simulink model "Example_IOBlock_Library_CCP"  (Simulink 10.3)
settings: Solver=FixedStepDiscrete  StartTime=0.0  StopTime=10.0  FixedStep=0.01  RelTol=1e-3
model workspace (MAT data in the model file):
  ParameterA_CCP_Test = Simulink.Parameter
  ParameterA_CCP_Test.Value = 23456
  ParameterA_CCP_Test.DataType = 'uint16'
  ParameterA_CCP_Test.Dimensions = [1 1]
  ParameterB_CCP_Test = Simulink.Parameter
  ParameterB_CCP_Test.Value = 0.5
  ParameterB_CCP_Test.DataType = 'single'
  ParameterB_CCP_Test.Min = 0
  ParameterB_CCP_Test.Max = 10
  ParameterB_CCP_Test.Dimensions = [1 1]
libraries: IOBlock_Library_TTC580 x9, AddOn_Lib_TTC580_CCP x2
settings Model: Creator=hokka  LastModifiedBy=hokka  MultithreadedSim=on
settings Model: SuppressorTable=|
  | <?xml version="1.0" encoding="UTF-8" standalone="yes" ?>
  | <!DOCTYPE boost_serialization>
  | <boost_serialization signature="serialization::archive" version="17">
  | <DiagnosticSuppressor class_id="0" tracking_level="0" version="7">
  | 	<Table class_id="1" tracking_level="0" version="0">
  | 		<count>7</count>
  | 		<bucket_count>8</bucket_count>
  | 		<item_version>0</item_version>
  | 		<item class_id="2" tracking_level="0" version="0">
  | 			<first class_id="3" tracking_level="0" version="7">
  | 				<Source class_id="4" tracking_level="0" version="0">
  | 					<count>1</count>
  | 					<item_version>0</item_version>
  | 					<item>74:2245</item>
  | 				</Source>
  | 			</first>
  | 			<second class_id="5" tracking_level="0" version="7">
  | 				<SuppressedData class_id="6" tracking_level="0" version="0">
  | 					<count>2</count>
  | 					<bucket_count>8</bucket_count>
  | 					<item_version>0</item_version>
  | 					<item class_id="7" tracking_level="0" version="0">
  | 						<first class_id="8" tracking_level="0" version="7">
  | 							<ID>Simulink:DataType:WarningOverFlowDetected</ID>
  | 							<Cause>
  | 								<Source>
  | 									<count>0</count>
  | 									<item_version>0</item_version>
  | 								</Source>
  | 							</Cause>
  | 						</first>
  | 						<second class_id="9" tracking_level="0" version="7">
  | 							<Comment></Comment>
  | 							<User></User>
  | 							<LastModified class_id="10" tracking_level="0" version="0">
  | 								<ptime_date class_id="11" tracking_level="0" version="0">
  | 									<date>20160608</date>
  | 								</ptime_date>
  | 								<ptime_time_duration class_id="12" tracking_level="0" version="1">
  | 									<is_special>0</is_special>
  | 									<time_duration_hours>15</time_duration_hours>
  | 									<time_duration_minutes>23</time_duration_minutes>
  | 									<time_duration_seconds>17</time_duration_seconds>
  | 									<time_duration_fractional_seconds>0</time_duration_fractional_seconds>
  | 								</ptime_time_duration>
  | 							</LastModified>
  | 							<SuppressionType>1</SuppressionType>
  | 						</second>
  | 					</item>
  | 					<item>
  | 						<first>
  | 							<ID>SimulinkFixedPoint:util:Overflowoccurred</ID>
  | 							<Cause>
  | 								<Source>
  | 									<count>0</count>
  | 									<item_version>0</item_version>
  | 								</Source>
  | 							</Cause>
  | 						</first>
  | 						<second>
  | 							<Comment></Comment>
  | 							<User></User>
  | 							<LastModified>
  | 								<ptime_date>
  | 									<date>20160608</date>
  | 								</ptime_date>
  | 								<ptime_time_duration>
  | 									<is_special>0</is_special>
  | 									<time_duration_hours>15</time_duration_hours>
  | 									<time_duration_minutes>23</time_duration_minutes>
  | 									<time_duration_seconds>17</time_duration_seconds>
  | 									<time_duration_fractional_seconds>0</time_duration_fractional_seconds>
  | 								</ptime_time_duration>
  | 							</LastModified>
  | 							<SuppressionType>1</SuppressionType>
  | 						</second>
  | 					</item>
  | 				</SuppressedData>
  | 			</second>
  | 		</item>
  | 		<item>
  | 			<first>
  | 				<Source>
  | 					<count>1</count>
  | 					<item_version>0</item_version>
  | 					<item>38:2245</item>
  | 				</Source>
  | 			</first>
  | 			<second>
  | 				<SuppressedData>
  | 					<count>2</count>
  | 					<bucket_count>8</bucket_count>
  | 					<item_version>0</item_version>
  | 					<item>
  | 						<first>
  | 							<ID>Simulink:DataType:WarningOverFlowDetected</ID>
  | 							<Cause>
  | 								<Source>
  | 									<count>0</count>
  | 									<item_version>0</item_version>
  | 								</Source>
  | 							</Cause>
  | 						</first>
  | 						<second>
  | 							<Comment></Comment>
  | 							<User></User>
  | 							<LastModified>
  | 								<ptime_date>
  | 									<date>20160608</date>
  | 								</ptime_date>
  | 								<ptime_time_duration>
  | 									<is_special>0</is_special>
  | 									<time_duration_hours>15</time_duration_hours>
  | 									<time_duration_minutes>23</time_duration_minutes>
  | 									<time_duration_seconds>17</time_duration_seconds>
  | 									<time_duration_fractional_seconds>0</time_duration_fractional_seconds>
  | 								</ptime_time_duration>
  | 							</LastModified>
  | 							<SuppressionType>1</SuppressionType>
  | 						</second>
  | 					</item>
  | 					<item>
  | 						<first>
  | 							<ID>SimulinkFixedPoint:util:Overflowoccurred</ID>
  | 							<Cause>
  | 								<Source>
  | 									<count>0</count>
  | 									<item_version>0</item_version>
  | 								</Source>
  | 							</Cause>
  | 						</first>
  | 						<second>
  | 							<Comment></Comment>
  | 							<User></User>
  | 							<LastModified>
  | 								<ptime_date>
  | 									<date>20160608</date>
  | 								</ptime_date>
  | 								<ptime_time_duration>
  | 									<is_special>0</is_special>
  | 									<time_duration_hours>15</time_duration_hours>
  | 									<time_duration_minutes>23</time_duration_minutes>
  | 									<time_duration_seconds>17</time_duration_seconds>
  | 									<time_duration_fractional_seconds>0</time_duration_fractional_seconds>
  | 								</ptime_time_duration>
  | 							</LastModified>
  | 							<SuppressionType>1</SuppressionType>
  | 						</second>
  | 					</item>
  | 				</SuppressedData>
  | 			</second>
  | 		</item>
  | 		<item>
  | 			<first>
  | 				<Source>
  | 					<count>1</count>
  | 					<item_version>0</item_version>
  | 					<item>23:2245</item>
  | 				</Source>
  | 			</first>
  | 			<second>
  | 				<SuppressedData>
  | 					<count>2</count>
  | 					<bucket_count>8</bucket_count>
  | 					<item_version>0</item_version>
  | 					<item>
  | 						<first>
  | 							<ID>Simulink:DataType:WarningOverFlowDetected</ID>
  | 							<Cause>
  | 								<Source>
  | 									<count>0</count>
  | 									<item_version>0</item_version>
  | 								</Source>
  | 							</Cause>
  | 						</first>
  | 						<second>
  | 							<Comment></Comment>
  | 							<User></User>
  | 							<LastModified>
  | 								<ptime_date>
  | 									<date>20160608</date>
  | 								</ptime_date>
  | 								<ptime_time_duration>
  | 									<is_special>0</is_special>
  | 									<time_duration_hours>15</time_duration_hours>
  | 									<time_duration_minutes>23</time_duration_minutes>
  | 									<time_duration_seconds>17</time_duration_seconds>
  | 									<time_duration_fractional_seconds>0</time_duration_fractional_seconds>
  | 								</ptime_time_duration>
  | 							</LastModified>
  | 							<SuppressionType>1</SuppressionType>
  | 						</second>
  | 					</item>
  | 					<item>
  | 						<first>
  | 							<ID>SimulinkFixedPoint:util:Overflowoccurred</ID>
  | 							<Cause>
  | 								<Source>
  | 									<count>0</count>
  | 									<item_version>0</item_version>
  | 								</Source>
  | 							</Cause>
  | 						</first>
  | 						<second>
  | 							<Comment></Comment>
  | 							<User></User>
  | 							<LastModified>
  | 								<ptime_date>
  | 									<date>20160608</date>
  | 								</ptime_date>
  | 								<ptime_time_duration>
  | 									<is_special>0</is_special>
  | 									<time_duration_hours>15</time_duration_hours>
  | 									<time_duration_minutes>23</time_duration_minutes>
  | 									<time_duration_seconds>17</time_duration_seconds>
  | 									<time_duration_fractional_seconds>0</time_duration_fractional_seconds>
  | 								</ptime_time_duration>
  | 							</LastModified>
  | 							<SuppressionType>1</SuppressionType>
  | 						</second>
  | 					</item>
  | 				</SuppressedData>
  | 			</second>
  | 		</item>
  | 		<item>
  | 			<first>
  | 				<Source>
  | 					<count>1</count>
  | 					<item_version>0</item_version>
  | 					<item>39:2245</item>
  | 				</Source>
  | 			</first>
  | 			<second>
  | 				<SuppressedData>
  | 					<count>2</count>
  | 					<bucket_count>8</bucket_count>
  | 					<item_version>0</item_version>
  | 					<item>
  | 						<first>
  | 							<ID>Simulink:DataType:WarningOverFlowDetected</ID>
  | 							<Cause>
  | 								<Source>
  | 									<count>0</count>
  | 									<item_version>0</item_version>
  | 								</Source>
  | 							</Cause>
  | 						</first>
  | 						<second>
  | 							<Comment></Comment>
  | 							<User></User>
  | 							<LastModified>
  | 								<ptime_date>
  | 									<date>20160608</date>
  | 								</ptime_date>
  | 								<ptime_time_duration>
  | 									<is_special>0</is_special>
  | 									<time_duration_hours>15</time_duration_hours>
  | 									<time_duration_minutes>23</time_duration_minutes>
  | 									<time_duration_seconds>17</time_duration_seconds>
  | 									<time_duration_fractional_seconds>0</time_duration_fractional_seconds>
  | 								</ptime_time_duration>
  | 							</LastModified>
  | 							<SuppressionType>1</SuppressionType>
  | 						</second>
  | 					</item>
  | 					<item>
  | 						<first>
  | 							<ID>SimulinkFixedPoint:util:Overflowoccurred</ID>
  | 							<Cause>
  | 								<Source>
  | 									<count>0</count>
  | 									<item_version>0</item_version>
  | 								</Source>
  | 							</Cause>
  | 						</first>
  | 						<second>
  | 							<Comment></Comment>
  | 							<User></User>
  | 							<LastModified>
  | 								<ptime_date>
  | 									<date>20160608</date>
  | 								</ptime_date>
  | 								<ptime_time_duration>
  | 									<is_special>0</is_special>
  | 									<time_duration_hours>15</time_duration_hours>
  | 									<time_duration_minutes>23</time_duration_minutes>
  | 									<time_duration_seconds>17</time_duration_seconds>
  | 									<time_duration_fractional_seconds>0</time_duration_fractional_seconds>
  | 								</ptime_time_duration>
  | 							</LastModified>
  | 							<SuppressionType>1</SuppressionType>
  | 						</second>
  | 					</item>
  | 				</SuppressedData>
  | 			</second>
  | 		</item>
  | 		<item>
  | 			<first>
  | 				<Source>
  | 					<count>1</count>
  | 					<item_version>0</item_version>
  | 					<item>103:2245</item>
  | 				</Source>
  | 			</first>
  | 			<second>
  | 				<SuppressedData>
  | 					<count>2</count>
  | 					<bucket_count>8</bucket_count>
  | 					<item_version>0</item_version>
  | 					<item>
  | 						<first>
  | 							<ID>Simulink:DataType:WarningOverFlowDetected</ID>
  | 							<Cause>
  | 								<Source>
  | 									<count>0</count>
  | 									<item_version>0</item_version>
  | 								</Source>
  | 							</Cause>
  | 						</first>
  | 						<second>
  | 							<Comment></Comment>
  | 							<User></User>
  | 							<LastModified>
  | 								<ptime_date>
  | 									<date>20160608</date>
  | 								</ptime_date>
  | 								<ptime_time_duration>
  | 									<is_special>0</is_special>
  | 									<time_duration_hours>15</time_duration_hours>
  | 									<time_duration_minutes>23</time_duration_minutes>
  | 									<time_duration_seconds>17</time_duration_seconds>
  | 									<time_duration_fractional_seconds>0</time_duration_fractional_seconds>
  | 								</ptime_time_duration>
  | 							</LastModified>
  | 							<SuppressionType>1</SuppressionType>
  | 						</second>
  | 					</item>
  | 					<item>
  | 						<first>
  | 							<ID>SimulinkFixedPoint:util:Overflowoccurred</ID>
  | 							<Cause>
  | 								<Source>
  | 									<count>0</count>
  | 									<item_version>0</item_version>
  | 								</Source>
  | 							</Cause>
  | 						</first>
  | 						<second>
  | 							<Comment></Comment>
  | 							<User></User>
  | 							<LastModified>
  | 								<ptime_date>
  | 									<date>20160608</date>
  | 								</ptime_date>
  | 								<ptime_time_duration>
  | 									<is_special>0</is_special>
  | 									<time_duration_hours>15</time_duration_hours>
  | 									<time_duration_minutes>23</time_duration_minutes>
  | 									<time_duration_seconds>17</time_duration_seconds>
  | 									<time_duration_fractional_seconds>0</time_duration_fractional_seconds>
  | 								</ptime_time_duration>
  | 							</LastModified>
  | 							<SuppressionType>1</SuppressionType>
  | 						</second>
  | 					</item>
  | 				</SuppressedData>
  | 			</second>
  | 		</item>
  | 		<item>
  | 			<first>
  | 				<Source>
  | 					<count>1</count>
  | 					<item_version>0</item_version>
  | 					<item>40:2245</item>
  | 				</Source>
  | 			</first>
  | 			<second>
  | 				<SuppressedData>
  | 					<count>2</count>
  | 					<bucket_count>8</bucket_count>
  | 					<item_version>0</item_version>
  | 					<item>
  | 						<first>
  | 							<ID>Simulink:DataType:WarningOverFlowDetected</ID>
  | 							<Cause>
  | 								<Source>
  | 									<count>0</count>
  | 									<item_version>0</item_version>
  | 								</Source>
  | 							</Cause>
  | 						</first>
  | 						<second>
  | 							<Comment></Comment>
  | 							<User></User>
  | 							<LastModified>
  | 								<ptime_date>
  | 									<date>20160608</date>
  | 								</ptime_date>
  | 								<ptime_time_duration>
  | 									<is_special>0</is_special>
  | 									<time_duration_hours>15</time_duration_hours>
  | 									<time_duration_minutes>23</time_duration_minutes>
  | 									<time_duration_seconds>17</time_duration_seconds>
  | 									<time_duration_fractional_seconds>0</time_duration_fractional_seconds>
  | 								</ptime_time_duration>
  | 							</LastModified>
  | 							<SuppressionType>1</SuppressionType>
  | 						</second>
  | 					</item>
  | 					<item>
  | 						<first>
  | 							<ID>SimulinkFixedPoint:util:Overflowoccurred</ID>
  | 							<Cause>
  | 								<Source>
  | 									<count>0</count>
  | 									<item_version>0</item_version>
  | 								</Source>
  | 							</Cause>
  | 						</first>
  | 						<second>
  | 							<Comment></Comment>
  | 							<User></User>
  | 							<LastModified>
  | 								<ptime_date>
  | 									<date>20160608</date>
  | 								</ptime_date>
  | 								<ptime_time_duration>
  | 									<is_special>0</is_special>
  | 									<time_duration_hours>15</time_duration_hours>
  | 									<time_duration_minutes>23</time_duration_minutes>
  | 									<time_duration_seconds>17</time_duration_seconds>
  | 									<time_duration_fractional_seconds>0</time_duration_fractional_seconds>
  | 								</ptime_time_duration>
  | 							</LastModified>
  | 							<SuppressionType>1</SuppressionType>
  | 						</second>
  | 					</item>
  | 				</SuppressedData>
  | 			</second>
  | 		</item>
  | 		<item>
  | 			<first>
  | 				<Source>
  | 					<count>1</count>
  | 					<item_version>0</item_version>
  | 					<item>36:2245</item>
  | 				</Source>
  | 			</first>
  | 			<second>
  | 				<SuppressedData>
  | 					<count>2</count>
  | 					<bucket_count>8</bucket_count>
  | 					<item_version>0</item_version>
  | 					<item>
  | 						<first>
  | 							<ID>Simulink:DataType:WarningOverFlowDetected</ID>
  | 							<Cause>
  | 								<Source>
  | 									<count>0</count>
  | 									<item_version>0</item_version>
  | 								</Source>
  | 							</Cause>
  | 						</first>
  | 						<second>
  | 							<Comment></Comment>
  | 							<User></User>
  | 							<LastModified>
  | 								<ptime_date>
  | 									<date>20160608</date>
  | 								</ptime_date>
  | 								<ptime_time_duration>
  | 									<is_special>0</is_special>
  | 									<time_duration_hours>15</time_duration_hours>
  | 									<time_duration_minutes>23</time_duration_minutes>
  | 									<time_duration_seconds>17</time_duration_seconds>
  | 									<time_duration_fractional_seconds>0</time_duration_fractional_seconds>
  | 								</ptime_time_duration>
  | 							</LastModified>
  | 							<SuppressionType>1</SuppressionType>
  | 						</second>
  | 					</item>
  | 					<item>
  | 						<first>
  | 							<ID>SimulinkFixedPoint:util:Overflowoccurred</ID>
  | 							<Cause>
  | 								<Source>
  | 									<count>0</count>
  | 									<item_version>0</item_version>
  | 								</Source>
  | 							</Cause>
  | 						</first>
  | 						<second>
  | 							<Comment></Comment>
  | 							<User></User>
  | 							<LastModified>
  | 								<ptime_date>
  | 									<date>20160608</date>
  | 								</ptime_date>
  | 								<ptime_time_duration>
  | 									<is_special>0</is_special>
  | 									<time_duration_hours>15</time_duration_hours>
  | 									<time_duration_minutes>23</time_duration_minutes>
  | 									<time_duration_seconds>17</time_duration_seconds>
  | 									<time_duration_fractional_seconds>0</time_duration_fractional_seconds>
  | 								</ptime_time_duration>
  | 							</LastModified>
  | 							<SuppressionType>1</SuppressionType>
  | 						</second>
  | 					</item>
  | 				</SuppressedData>
  | 			</second>
  | 		</item>
  | 	</Table>
  | </DiagnosticSuppressor>
  | 
  | </boost_serialization>
  | 
  | </boost_serialization>
settings DataIOCC: LimitDataPoints=on
settings OptimizationCC: InitFltsAndDblsToZero=on  LifeSpan=1  EfficientTunableParamExpr=on
settings DebuggingCC: SolverPrmCheckMsg=warning  InheritedTsInSrcMsg=none
settings HardwareCC: ProdLargestAtomicInteger=Long  ProdLargestAtomicFloat=Double  ProdIntDivRoundTo=Zero  ProdEndianess=BigEndian  ProdHWDeviceType=Texas Instruments->TMS570 Cortex-R4  TargetIntDivRoundTo=Zero  TargetEndianess=BigEndian  TargetHWDeviceType=Generic->32-bit Embedded Processor
settings SFSimCC: MATLABDynamicMemAlloc=off
settings RTWCC: Description=Real-Time Workshop Embedded Coder (no auto configuration)  SystemTargetFile=ert.tlc  GenCodeOnly=on  TemplateMakefile=ert_TTC580.tmf
settings CodeAppCC: IgnoreCustomStorageClasses=off  CustomSymbolStrType=$N$R$M  InternalIdentifier=Classic
settings ERTTargetCC: MultiwordLength=2048  SupportAbsoluteTime=off  SupportNonFinite=off  GenerateASAP2=on  ERTCustomFileTemplate=example_file_process.tlc  ConvertIfToSwitch=off  SuppressUnreachableDefaultCases=off
settings ConfigComp: CovSFcnEnable=off

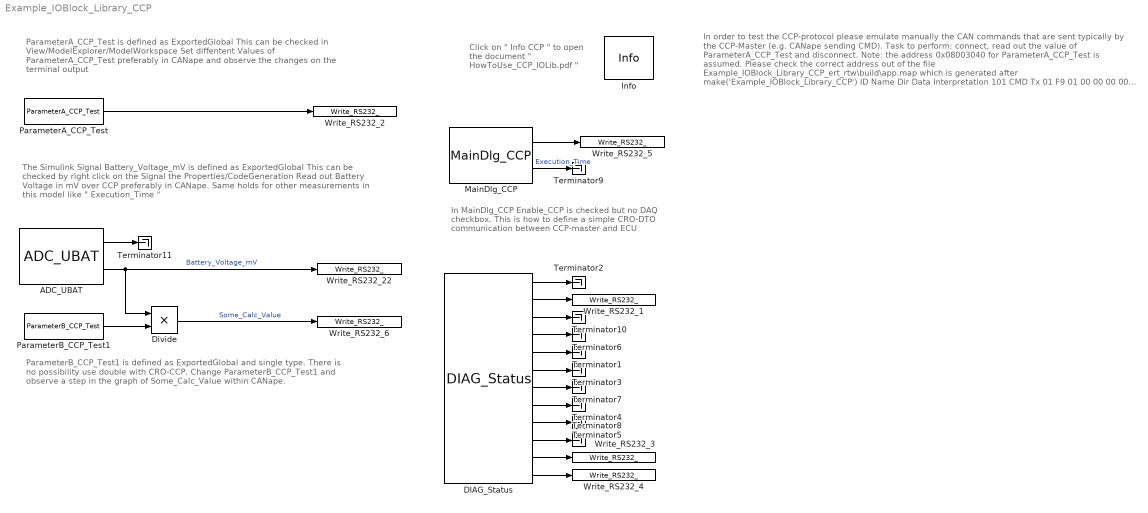
== system Example_IOBlock_Library_CCP ==
  note: In order to test the CCP-protocol please emulate manually the CAN commands that are sent typically by the CCP-Master (e.g. CANape sending CMD).
      |
      | Task to perform: connect, read out the value of ParameterA_CCP_Test and disconnect.
      |
      | Note: the address 0x08003040 for ParameterA_CCP_Test is assumed. Please check the correct address out of
      | the file Example_IOBlock_Library_CCP_ert_rtw\build\app.map which is generated after make('Example_IOBlock_Library_CCP')
      |
      | ID	Name	       Dir	Data	                Interpretation
      | 101	CMD		Tx	01 F9 01 00 00 00 00 00	CONNECT addr=0001h (CCP station addr.)
      | 102	RES		Rx	FF 00 F9 00 01 00 00 00	Ok:CONNECT
      | 101	CMD		Tx	17 FA 00 00 00 00 00 00	EXCHANGE_ID
      | 102	RES		Rx	FF 00 FA 08 00 01 00 8E	Ok:EXCHANGE_ID size=8 type=00h avail=01h protect=00h
      | 101	CMD		Tx	1B FB 02 01 00 00 00 00	GET_CCP_VERSION version=02h release=01h
      | 102	RES		Rx	FF 00 FB 02 01 01 00 8E	Ok:GET_CCP_VERSION version=02h release=01h
      | 101	CMD		Tx	0F FC 02 00 08 00 30 40	SHORT_UPLOAD size=2 ext=00h addr=08003040h
      | 102	RES		Rx	FF 00 FC 5B A0 01 00 8E	Ok:SHORT_UPLOAD data=5Bh A0h (decimal value=23456)
      | 101	CMD		Tx	07 FD 01 01 00 00  00 00	DISCONNECT addr=0001h (CCP station addr)
      | 102	RES		Rx	FF 00 FD  xx xx xx xx xx	Ok:DISCONNECT
  note: In MainDlg_CCP Enable_CCP is checked but no DAQ checkbox. This is how to define a simple CRO-DTO communication between CCP-master and ECU
  note: ParameterA_CCP_Test is defined as ExportedGlobal
      | This can be checked in View/ModelExplorer/ModelWorkspace
      | Set diffentent Values of ParameterA_CCP_Test preferably in CANape
      | and observe the changes on the terminal output
  note: The Simulink Signal Battery_Voltage_mV is defined as ExportedGlobal
      | This can be checked by right click on the Signal the Properties/CodeGeneration
      | Read out Battery Voltage in mV over CCP preferably in CANape.
      | Same holds for other measurements in this model like " Execution_Time "
  note: ParameterB_CCP_Test1 is defined as ExportedGlobal and single type.
      | There is no possibility use double with CRO-CCP.
      | Change ParameterB_CCP_Test1 and observe a step in the graph of Some_Calc_Value within CANape.
  note: Click on " Info CCP " to
      | open the document
      | " HowToUse_CCP_IOLib.pdf "
  ADC_UBAT : IOBlock_Library_TTC580/ADC Blocks TTC580 IOlib/ADC_UBAT  SampleTime=-1  ttlib=IO_Blk_Lib_TTC500  ttDescription=ADC_UBAT  tt_iolib_version=0.26  adc_channel=IO_ADC_UBAT  adc_type=IO_ADC_ABSOLUTE  range=IO_ADC_RANGE_32V  pupd=IO_ADC_NO_PULL  sensor_supply=IO_PIN_NONE
      settings: SourceProductName=I/O Blocklibrary for TTC580
  DIAG_Status : IOBlock_Library_TTC580/System  Blocks TTC580 IOlib/DIAG_Status  Priority=-10  SampleTime=-1  ttlib=IO_Blk_Lib_TTC500  ttDescription=DIAG_Status  tt_iolib_version=0.16  FPGA_Major=16  FPGA_Minor=5  IODriver_Major=2  IODriver_Minor=14
      settings: SourceProductName=I/O Blocklibrary for TTC580
  Divide : Product  Inputs=**  OutDataTypeStr=single
  Info : AddOn_Lib_TTC580_CCP/Examples/Info  bla=0
      settings: SourceProductName=Addon (CCP) for I/O Blocklib TTC580
  MainDlg_CCP : AddOn_Lib_TTC580_CCP/System  Blocks TTC580 Addon-IOlib/MainDlg_CCP  SampleTime=-1  ttlib=IO_Blk_Lib_TTC500  ttDescription=MainDlg_CCP  tt_iolib_version=0.25  baudrate_CAN0=500  tseg1_CAN0=6  tseg2_CAN0=2  sjw_CAN0=1  brp_CAN0=1  baudrate_CAN1=500  tseg1_CAN1=6  tseg2_CAN1=2  sjw_CAN1=1  brp_CAN1=1  baudrate_CAN2=500  tseg1_CAN2=6  tseg2_CAN2=2  sjw_CAN2=1  brp_CAN2=1  baudrate_CAN3=500  baudrate_CAN4=500  baudrate_CAN5=500  baudrate_CAN6=500  tseg1=6  tseg2=2  sjw=1  Duration_ms=10  glitch_filter_time=180  watchdog_window_size=SAFETY_CONF_WINDOW_SIZE_100_PERCENT  watchdog_reset_behavior=SAFETY_CONF_RESETS_DISABLED  brp=0  Enable_sending_DM1_of_J1939=off  DM1_Channel=IO_CAN_CHANNEL_0  J1939SorceAddress=0  DM2_Basis_Address=63488  Show_version_information=off  Major_Number=0  Minor_Number=1  Revison_Number=1  Node_Number=1  Enable_Reset_by_TTCDownloader=on  bFlashOverEthernet=off  Enable_CCP=on  CRO_ID=hex2dec('101')  DTO_ID=hex2dec('102')  CCP_Station_Addr_raw=1  CCP_Station_ID=ECU00001  CPP_channel=IO_CAN_CHANNEL_0  CPP_id_format=IO_CAN_STD_FRAME  bEnable_DAQ0=off  bEnable_DAQ1_2=off  ODT_total=10  bEnable_ErrorCBAction=off  bDIAG_ERR_DISABLE_SSW0=off  bDIAG_ERR_DISABLE_SSW1=off  bDIAG_ERR_DISABLE_SSW2=off
      settings: SourceProductName=Addon (CCP) for I/O Blocklib TTC580
  ParameterA_CCP_Test : Constant  Value=ParameterA_CCP_Test  OutDataTypeStr=uint16
  ParameterB_CCP_Test1 : Constant  Value=ParameterB_CCP_Test  OutDataTypeStr=single
  Terminator{1..11} (11 alike) : Terminator
  Write_RS232_1 : IOBlock_Library_TTC580/UART TTC580 IOlib/Write_RS232_  Priority=1  SampleTime=-1  ttlib=IO_Blk_Lib_TTC500  ttDescription=Write_RS232_  tt_iolib_version=0.25  Comment=diag_state =
      settings: SourceProductName=I/O Blocklibrary for TTC580
  Write_RS232_2 : IOBlock_Library_TTC580/UART TTC580 IOlib/Write_RS232_  Priority=18  SampleTime=-1  ttlib=IO_Blk_Lib_TTC500  ttDescription=Write_RS232_  tt_iolib_version=0.25  Comment=ParameterA_CCP_Test =
      settings: SourceProductName=I/O Blocklibrary for TTC580
  Write_RS232_22 : IOBlock_Library_TTC580/UART TTC580 IOlib/Write_RS232_  Priority=17  SampleTime=-1  ttlib=IO_Blk_Lib_TTC500  ttDescription=Write_RS232_  tt_iolib_version=0.25  Comment=Value ADC_UBAT (mV)=
      settings: SourceProductName=I/O Blocklibrary for TTC580
  Write_RS232_3 : IOBlock_Library_TTC580/UART TTC580 IOlib/Write_RS232_  Priority=9  SampleTime=-1  ttlib=IO_Blk_Lib_TTC500  ttDescription=Write_RS232_  tt_iolib_version=0.25  Comment=b_FPGA_version_OK =
      settings: SourceProductName=I/O Blocklibrary for TTC580
  Write_RS232_4 : IOBlock_Library_TTC580/UART TTC580 IOlib/Write_RS232_  Priority=9  SampleTime=-1  ttlib=IO_Blk_Lib_TTC500  ttDescription=Write_RS232_  tt_iolib_version=0.25  Comment=b_IODrv_version_OK =
      settings: SourceProductName=I/O Blocklibrary for TTC580
  Write_RS232_5 : IOBlock_Library_TTC580/UART TTC580 IOlib/Write_RS232_  Priority=0  SampleTime=-1  ttlib=IO_Blk_Lib_TTC500  ttDescription=Write_RS232_  tt_iolib_version=0.25  Comment=ErrorCode MainDlg =
      settings: SourceProductName=I/O Blocklibrary for TTC580
  Write_RS232_6 : IOBlock_Library_TTC580/UART TTC580 IOlib/Write_RS232_  Priority=20  SampleTime=-1  ttlib=IO_Blk_Lib_TTC500  ttDescription=Write_RS232_  tt_iolib_version=0.25  Comment=Some_Calc_Value =
      settings: SourceProductName=I/O Blocklibrary for TTC580
  wires:
  DIAG_Status/2 -> Write_RS232_1/1
  DIAG_Status/3 -> Terminator10/1
  DIAG_Status/4 -> Terminator6/1
  DIAG_Status/5 -> Terminator1/1
  DIAG_Status/6 -> Terminator3/1
  DIAG_Status/7 -> Terminator7/1
  DIAG_Status/8 -> Terminator4/1
  DIAG_Status/9 -> Terminator5/1
  DIAG_Status/10 -> Terminator8/1
  DIAG_Status/1 -> Terminator2/1
  DIAG_Status/11 -> Write_RS232_3/1
  DIAG_Status/12 -> Write_RS232_4/1
  ADC_UBAT/1 -> Terminator11/1
  ADC_UBAT/2 -> Divide/1, Write_RS232_22/1  "Battery_Voltage_mV"
  MainDlg_CCP/2 -> Terminator9/1  "Execution_Time"
  MainDlg_CCP/1 -> Write_RS232_5/1
  ParameterA_CCP_Test/1 -> Write_RS232_2/1
  ParameterB_CCP_Test1/1 -> Divide/2
  Divide/1 -> Write_RS232_6/1  "Some_Calc_Value"
